simulink model "mpu6050 - Copy"  (R2017a)
settings: Solver=FixedStepDiscrete  StartTime=0.0  StopTime=inf  RelTol=1e-3
PostLoadFcn:
  | ChipSelect = 1;  % choose I2C comms
  | AddressAlt = 0;  % use default address
  | 
  | if AddressAlt == 1
  | % b1101001 (pin AD0 is logic high).
  | SlvAddr = uint8(bin2dec('1101001'));  % ADDR ALT = 1
  | else
  | % b1101000 (pin AD0 is logic low)
  | SlvAddr = uint8(bin2dec('1101000'));  % ADDR ALT = 0
  | end
  | SlvAddr = uint8(hex2dec('68'));
  | 
  | 
  | % 0x3B 59 ACCEL_XOUT[15:8]
  | % 0x3C 60 ACCEL_XOUT[7:0]
  | % 0x3D 61 ACCEL_YOUT[15:8]
  | % 0x3E 62 ACCEL_YOUT[7:0]
  | % 0x3F 63 ACCEL_ZOUT[15:8]
  | % 0x40 64 ACCEL_ZOUT[7:0]
  | 
  | AccelXRegAddr = uint8(hex2dec('3B'));
  | AccelYRegAddr = uint8(hex2dec('3D'));
  | AccelZRegAddr = uint8(hex2dec('3F'));
  | 
  | % 0x43 67 GYRO_XOUT[15:8]
  | % 0x44 68 GYRO_XOUT[7:0]
  | % 0x45 69 GYRO_YOUT[15:8]
  | % 0x46 70 GYRO_YOUT[7:0]
  | % 0x47 71 GYRO_ZOUT[15:8]
  | % 0x48 72 GYRO_ZOUT[7:0]
  | 
  | GyroXRegAddr = uint8(hex2dec('43'));
  | GyroYRegAddr = uint8(hex2dec('45'));
  | GyroZRegAddr = uint8(hex2dec('47'));
  | 
  | deviceAddr = fi(SlvAddr,0,7,0);
  | 
  | powerRegAddr = uint8(hex2dec('6B'));
  | powerRegData = bin2dec('10000001');
(part 4 of 4)

== stateflow chart mpu6050 - Copy/I2C_MPU6050_IP/MPU6050_Interface2 ==
  settings: executeAtInitialization=1
  note: I2C Configuration for MPU6050
  state init
    %initstate
    Valid_Out = 0;
    isDeviceSetup = 0;
    slv_addr = SlvAddr;
    %TODO delete all
    tmp = 0;
    tmpConfig = 0;
    tmpReadGyro = 0;
    tmpReadAccel = 0;
    tmpValid = 0;
    tmpReadDevice = 0;
    tmpHere = 0;
    tmpData = 128;
    gyroRes = 250.0/32768.0;
    accelRes = 2.0/32768.0;
  note: 0x3B 59 ACCEL_XOUT[15:8]
      | 0x3C 60 ACCEL_XOUT[7:0]
      | 0x3D 61 ACCEL_YOUT[15:8]
      | 0x3E 62 ACCEL_YOUT[7:0]
      | 0x3F 63 ACCEL_ZOUT[15:8]
      | 0x40 64 ACCEL_ZOUT[7:0]
      |
      | 0x43 67 GYRO_XOUT[15:8]
      | 0x44 68 GYRO_XOUT[7:0]
      | 0x45 69 GYRO_YOUT[15:8]
      | 0x46 70 GYRO_YOUT[7:0]
      | 0x47 71 GYRO_ZOUT[15:8]
      | 0x48 72 GYRO_ZOUT[7:0]
      |
      | 0x6B 107 PWR_MGMT_1
      | 0x6C 108 PWR_MGMT_2
  note: TODO check functions - dont need to convert?
  state idle
    %idlestate
    enb 	= 0;
    rw 		= 0;
    mode 	= 0;
    cnt      = 0;
    reg_byte_mode = 0;
    tmp = isDeviceSetup;
  state Configuration [group]
    state configurationStart
      %force success config
      isDeviceSetup = 0;
    state setupReadWhoAmI
      entry:
      enb = 1;
      rw = 1;
      mode = 0;
      reg_addr = 117;
    state waitforNotBusy0
      enb=0; tmpData=1;
    state readWhoAmI1
      %tmpData = uint8(data_in);
    state setupReadPwrMgmt1
      entry:
      enb = 1;
      rw = 1;
      mode = 0;
      reg_addr = 107;
    state waitforNotBusy1
      enb=0; tmpData=2;
    state setupWritePwrMgmt1
      enb = 1;
      rw = 0;
      mode = 0;
      reg_addr = 107; %0x6B
      data_out = 0;
    state readPwrManagement1
      tmpData = uint8(data_in);
    state waitforNotBusy2
      enb=0; %tmpData=3;
    state setupFS_SEL
      enb = 1;
      rw = 0;
      mode = 0;
      reg_addr = 27; %0x1b
      data_out = 16; %fs range +/- 1000
    state waitforNotBusy3
      enb=0; %tmpData=3;
    state configStartBiasLoop
      i = 0; biasSamples = 1000;
      GyroX = 0;  gyroXBias = 0;
      GyroY = 0;  gyroYBias = 0;
      GyroZ = 0;  gyroZBias = 0;
      AccelX = 0; accelXBias = 0;
      AccelY = 0; accelYBias = 0;
      AccelZ = 0; accelZBias = 0;
      gyroTmpBiasX = 0; gyroTmpBiasY = 0;
      gyroTmpBiasZ = 0;
      accelTmpBiasX = 0; accelTmpBiasY = 0;
      accelTmpBiasZ = 0;
      tmpHere = 1;
    state incrementBias
      i = sum_int16(i,1);
      accelTmpBiasX = sum_int16(accelTmpBiasX,AccelX);
      accelTmpBiasY = sum_int16(accelTmpBiasY,AccelY);
      accelTmpBiasZ = sum_int16(accelTmpBiasZ,AccelZ);
      gyroTmpBiasX  = sum_int16(gyroTmpBiasX, GyroX);
      gyroTmpBiasY  = sum_int16(gyroTmpBiasY, GyroY);
      gyroTmpBiasZ  = sum_int16(gyroTmpBiasZ, GyroZ);
    state configCalculateBiases
      accelXBias = divide_int16(accelTmpBiasX,biasSamples);
      accelYBias = divide_int16(accelTmpBiasY,biasSamples);
      %accelZBias = divide_int16(accelTmpBiasZ,biasSamples);
      gyroXBias  = divide_int16(gyroTmpBiasX, biasSamples);
      gyroYBias  = divide_int16(gyroTmpBiasY, biasSamples);
      %gyroZBias  = divide_int16(gyroTmpBiasZ, biasSamples);
    state cfgDone
      isDeviceSetup = 1;
      tmpConfig = 1;
      tmpHere = 0;
    configurationStart -> setupReadWhoAmI
    setupReadWhoAmI -> waitforNotBusy0 : [busy==1]
    waitforNotBusy0 -> readWhoAmI1 [order 2] : [mstr_ack==1]
    waitforNotBusy0 -> (junction 2445) [order 1] : [n_ack==1]
    readWhoAmI1 -> setupReadPwrMgmt1 : [busy==0]
    setupReadPwrMgmt1 -> Configuration.waitforNotBusy1 : [busy==1]
    Configuration.waitforNotBusy1 -> (junction 2445) [order 1] : [n_ack==1]
    Configuration.waitforNotBusy1 -> readPwrManagement1 [order 2] : [mstr_ack==1]
    readPwrManagement1 -> setupWritePwrMgmt1 : [busy==0]
    setupWritePwrMgmt1 -> waitforNotBusy2 : [busy==1]
    waitforNotBusy2 -> setupFS_SEL [order 1] : [busy==0]
    waitforNotBusy2 -> (junction 2445) [order 2] : [n_ack==1]
    setupFS_SEL -> waitforNotBusy3 : [busy==1]
    waitforNotBusy3 -> configStartBiasLoop : [busy==0]
    configStartBiasLoop -> incrementBias
    incrementBias -> configCalculateBiases [order 2]
    configCalculateBiases -> cfgDone
  state ReadDeviceData [group]
    note: DEVID is an example of
        | doing a 1-byte READ
    note: 0x75 117 - WHO_AM_I[6:1]
        | TODO
        |    THIS IS DEBUGGING ONLY DELETE!
    state getDEVID
      entry:
      enb = 1;
      rw = 1;
      mode = 0;
      reg_addr =   uint8(117);
      tmpReadDevice = 1;
    state waitforNotBusy1
      enb=0;
    state readDEVID
      deviceId = uint8(data_in);
    state waitforNotBusy6
      %
    state getRegData
      entry:
      enb = 1;
      rw = 1;
      mode = 0;
      reg_addr = userRegAddr;
    state waitforNotBusy5
      enb=0;
    state readUserRegData
      regdata = uint8(data_in);
    getDEVID -> ReadDeviceData.waitforNotBusy1 : [busy==1]
    ReadDeviceData.waitforNotBusy1 -> waitforNotBusy6 [order 2] : [n_ack==1]
    ReadDeviceData.waitforNotBusy1 -> readDEVID [order 1] : [mstr_ack==1]
    readDEVID -> getRegData : [busy==0]
    waitforNotBusy6 -> (junction 2281)
    getRegData -> waitforNotBusy5 : [busy==1]
    waitforNotBusy5 -> readUserRegData [order 1] : [mstr_ack==1]
    waitforNotBusy5 -> (junction 2281) [order 2] : [n_ack==1]
  state Valid
    en: enb = 0;
    cnt = 0;
    Valid_Out = 1;
    du: cnt = cnt + 1;
    tmpValid = 1;
  state check_cfg
    en: enb = 0;
    cnt = 0;
    du: cnt = cnt + 1;
    tmpCheckCng = 1
  state SetupBias [group] [commented out]
    state biasWritePwrMgmt1 [commented out]
      %reset device
      enb = 1;
      rw = 0;
      mode = 0;
      reg_addr = 107; %0x6B
      data_out = 128;
    state waitforNotBusyb [commented out]
      enb=0; i =0;
    state delay [commented out]
      i = i + 1;
    state biasWritePwrMgmt2 [commented out]
      enb = 1;
      rw = 0;
      mode = 0;
      reg_addr = 107; %0x6B
      data_out = 1;
    state waitforNotBusyb1 [commented out]
      enb=0; i =0;
    state biasWritePwrMgmt1_1 [commented out]
      enb = 1;
      rw = 0;
      mode = 0;
      reg_addr = 107; %0x6B
      data_out = 1;
    state waitforNotBusyb2 [commented out]
      enb=0; i =0;
    state delay1 [commented out]
      i = i + 1;
    state biasWriteIntEnable [commented out]
      %disable all interrupts
      enb = 1;
      rw = 0;
      mode = 0;
      reg_addr = 56;
      data_out = 00;
    state waitforNotBusyb3 [commented out]
      enb=0; i =0;
    state biasWriteFIFO [commented out]
      %disable FIFO
      enb = 1;
      rw = 0;
      mode = 0;
      reg_addr = 35;
      data_out = 00;
    state waitforNotBusyb4 [commented out]
      enb=0; i =0;
    state biasWritePwrMgmt1_2 [commented out]
      %turn on internal clk src
      enb = 1;
      rw = 0;
      mode = 0;
      reg_addr = 107;
      data_out = 00;
    state waitforNotBusyb5 [commented out]
      enb=0; i =0;
    state biasWriteI2cMstrCtrl [commented out]
      %disable i2c master
      enb = 1;
      rw = 0;
      mode = 0;
      reg_addr = 36;
      data_out = 00;
    state waitforNotBusyb6 [commented out]
      enb=0; i =0;
    state biasWriteUserCtrl [commented out]
      %disable FIFO & i2c maste
      enb = 1;
      rw = 0;
      mode = 0;
      reg_addr = 36;
      data_out = 00;
    state waitforNotBusyb7 [commented out]
      enb=0; i =0;
    state biasWriteUserCtrl1 [commented out]
      %reset FIFO & DMP
      enb = 1;
      rw = 0;
      mode = 0;
      reg_addr = 36;
      data_out = 12;
    state waitforNotBusyb8 [commented out]
      enb=0; i =0;
    state delay2 [commented out]
      i = i + 1;
    state biasWriteConfig [commented out]
      %set lowpassfilter to 188hz
      enb = 1;
      rw = 0;
      mode = 0;
      reg_addr = 26;
      data_out = 1;
    state waitforNotBusyb9 [commented out]
      enb=0; i =0;
    state biasWriteSmplrtDiv [commented out]
      %samplerate 1khz
      enb = 1;
      rw = 0;
      mode = 0;
      reg_addr = 36;
      data_out = 26;
    state waitforNotBusyb10 [commented out]
      enb=0; i =0;
    waitforNotBusyb -> (junction 2753) [commented out] : [n_ack==1]
    biasWritePwrMgmt1 -> waitforNotBusyb [commented out] : [busy==1]
    waitforNotBusyb -> delay [commented out] : [busy==0]
    delay -> delay [commented out] : [i < 100]
    delay -> biasWritePwrMgmt2 [commented out]
    waitforNotBusyb1 -> (junction 2753) [commented out] : [n_ack==1]
    biasWritePwrMgmt2 -> waitforNotBusyb1 [commented out] : [busy==1]
    waitforNotBusyb1 -> biasWritePwrMgmt1_1 [commented out] : [busy==0]
    waitforNotBusyb2 -> (junction 2753) [commented out] : [n_ack==1]
    waitforNotBusyb3 -> (junction 2753) [commented out] : [n_ack==1]
    (junction 2753) -> (junction 2832) [commented out]
    waitforNotBusyb4 -> (junction 2753) [commented out] : [n_ack==1]
    waitforNotBusyb5 -> (junction 2753) [commented out] : [n_ack==1]
    biasWritePwrMgmt1_1 -> waitforNotBusyb2 [commented out] : [busy==1]
    waitforNotBusyb2 -> delay1 [commented out] : [busy==0]
    delay1 -> biasWriteIntEnable [commented out]
    delay1 -> delay1 [commented out] : [i < 200]
    biasWriteIntEnable -> waitforNotBusyb3 [commented out] : [busy==1]
    waitforNotBusyb3 -> biasWriteFIFO [commented out] : [busy==0]
    biasWriteFIFO -> waitforNotBusyb4 [commented out] : [busy==1]
    waitforNotBusyb4 -> biasWritePwrMgmt1_2 [commented out] : [busy==0]
    biasWritePwrMgmt1_2 -> waitforNotBusyb5 [commented out] : [busy==1]
    waitforNotBusyb5 -> biasWriteI2cMstrCtrl [commented out] : [busy==0]
    waitforNotBusyb6 -> (junction 2834) [commented out] : [n_ack==1]
    waitforNotBusyb7 -> (junction 2834) [commented out] : [n_ack==1]
    waitforNotBusyb8 -> (junction 2834) [commented out] : [n_ack==1]
    (junction 2834) -> (junction 2832) [commented out]
    waitforNotBusyb9 -> (junction 2834) [commented out] : [n_ack==1]
    biasWriteI2cMstrCtrl -> waitforNotBusyb6 [commented out] : [busy==1]
    waitforNotBusyb6 -> biasWriteUserCtrl [commented out] : [busy==0]
    biasWriteUserCtrl -> waitforNotBusyb7 [commented out] : [busy==1]
    waitforNotBusyb7 -> biasWriteUserCtrl1 [commented out] : [busy==0]
    (junction 2869) -> (junction 2832) [commented out]
    biasWriteUserCtrl1 -> waitforNotBusyb8 [commented out] : [busy==1]
    waitforNotBusyb8 -> delay2 [commented out] : [busy==0]
    delay2 -> delay2 [commented out] : [i < 200]
    delay2 -> biasWriteConfig [commented out]
    biasWriteConfig -> waitforNotBusyb9 [commented out] : [busy==1]
    waitforNotBusyb9 -> biasWriteSmplrtDiv [commented out] : [busy==0]
    biasWriteSmplrtDiv -> waitforNotBusyb10 [commented out] : [busy==1]
    waitforNotBusyb10 -> (junction 2869) [commented out] : [n_ack==1]
    waitforNotBusyb10 -> ? [commented out] : [busy==0]
  state ReadAccelData [group]
    state setupReadAccelXoutH
      entry:
      enb = 1;
      rw = 1;
      mode = 0;
      reg_addr = 59; %0x3b
      tmpReadAccel = 1;
    state waitforNotBusya1
      enb=0; tmpData = 1;
    state readAccelXoutH
      tempVal = uint8(data_in);
      tmpData = 2;
    state setupReadAccelXoutL
      entry:
      enb = 1;
      rw = 1;
      mode = 0;
      reg_addr = 60; %0x3c
    state waitforNotBusya3
      enb=0; tmpData = 2;
    state readAccelXoutL
      AccelX = convert_int16(tempVal, data_in);
      AccelX = subtract_int16(AccelX,accelXBias);
    state setupReadAccelYoutH
      entry:
      enb = 1;
      rw = 1;
      mode = 0;
      reg_addr = 61; %0x3d
    state waitforNotBusya4
      enb=0; tmpData = 3;
    state readAccelYoutH
      tempVal = uint8(data_in);
    state setupReadAccelYoutL
      entry:
      enb = 1;
      rw = 1;
      mode = 0;
      reg_addr = 62; %0x3e
    state waitforNotBusya5
      enb=0;tmpData = 4;
    state readGyroYoutL
      AccelY = convert_int16(tempVal, data_in)
      AccelY = subtract_int16(AccelY,accelYBias);;
    state setupReadAccelZoutH
      entry:
      enb = 1;
      rw = 1;
      mode = 0;
      reg_addr = 63; %0x3f
    state waitforNotBusya6
      enb=0;tmpData = 5;
    state readAccelZoutH
      tempVal = uint8(data_in);
    state setupReadAccelZoutL
      entry:
      enb = 1;
      rw = 1;
      mode = 0;
      reg_addr = 64; %0x40
    state waitforNotBusya7
      enb=0;tmpData = 6;
    state readAccelZoutL
      AccelZ = convert_int16(tempVal, data_in);
      %AccelZ = subtract_int16(AccelZ,accelZBias);
    setupReadAccelXoutH -> waitforNotBusya1 : [busy==1]
    waitforNotBusya1 -> (junction 2534) [order 2] : [n_ack==1]
    waitforNotBusya1 -> readAccelXoutH [order 1] : [mstr_ack==1]
    readAccelXoutH -> setupReadAccelXoutL : [busy==0]
    setupReadAccelXoutL -> waitforNotBusya3 : [busy==1]
    waitforNotBusya3 -> (junction 2534) [order 2] : [n_ack==1]
    waitforNotBusya3 -> readAccelXoutL [order 1] : [mstr_ack==1]
    readAccelXoutL -> setupReadAccelYoutH : [busy==0]
    waitforNotBusya4 -> (junction 2534) [order 2] : [n_ack==1]
    waitforNotBusya5 -> (junction 2534) [order 2] : [n_ack==1]
    waitforNotBusya6 -> (junction 2534) [order 2] : [n_ack==1]
    waitforNotBusya7 -> (junction 2534) [order 2] : [n_ack==1]
    setupReadAccelYoutH -> waitforNotBusya4 : [busy==1]
    waitforNotBusya4 -> readAccelYoutH [order 1] : [mstr_ack==1]
    readAccelYoutH -> setupReadAccelYoutL : [busy==0]
    setupReadAccelYoutL -> waitforNotBusya5 : [busy==1]
    waitforNotBusya5 -> ReadAccelData.readGyroYoutL [order 1] : [mstr_ack==1]
    ReadAccelData.readGyroYoutL -> setupReadAccelZoutH : [busy==0]
    setupReadAccelZoutH -> waitforNotBusya6 : [busy==1]
    waitforNotBusya6 -> readAccelZoutH [order 1] : [mstr_ack==1]
    readAccelZoutH -> setupReadAccelZoutL : [busy==0]
    setupReadAccelZoutL -> waitforNotBusya7 : [busy==1]
    waitforNotBusya7 -> readAccelZoutL [order 1] : [mstr_ack==1]
  state ReadGyroData [group]
    state setupReadGyroXoutH
      entry:
      enb = 1;
      rw = 1;
      mode = 0;
      reg_addr = 67; %0x43
      tmpReadGyro = 1;
    state waitforNotBusy06
      enb=0;tmpData = 10;
    state readGyroXoutH
      tempVal = uint8(data_in);
    state setupReadGyroXoutL
      entry:
      enb = 1;
      rw = 1;
      mode = 0;
      reg_addr = 68; %0x44
    state waitforNotBusy07
      enb=0;tmpData = 11;
    state readGyroXoutL
      GyroX = convert_int16(tempVal, data_in);
      GyroX = subtract_int16(GyroX,gyroXBias);
    state setupReadGyroYoutH
      entry:
      enb = 1;
      rw = 1;
      mode = 0;
      reg_addr = 69; %0x45
    state waitforNotBusy04
      enb=0;tmpData = 12;
    state readGyroYoutH
      tempVal = uint8(data_in);
    state setupReadGyroYoutL
      entry:
      enb = 1;
      rw = 1;
      mode = 0;
      reg_addr = 70; %0x46
    state waitforNotBusy05
      enb=0;tmpData = 13;
    state readGyroYoutL
      GyroY = convert_int16(tempVal, data_in);
      GyroY = subtract_int16(GyroY,gyroYBias);
    state setupReadGyroZoutH
      entry:
      enb = 1;
      rw = 1;
      mode = 0;
      reg_addr = 71; %0x47
    state waitforNotBusy01
      enb=0;tmpData = 14;
    state readGyroZoutH
      tempVal = uint8(data_in);
    state setupReadGyroZoutL
      entry:
      enb = 1;
      rw = 1;
      mode = 0;
      reg_addr = 72; %0x48
    state waitforNotBusy03
      enb=0;tmpData = 15;
    state readGyroZoutL
      GyroZ = convert_int16(tempVal, data_in);
      %GyroZ = subtract_int16(GyroZ,gyroZBias);
    setupReadGyroXoutH -> waitforNotBusy06 : [busy==1]
    waitforNotBusy06 -> (junction 2595) [order 2] : [n_ack==1]
    waitforNotBusy06 -> readGyroXoutH [order 1] : [mstr_ack==1]
    readGyroXoutH -> setupReadGyroXoutL : [busy==0]
    setupReadGyroXoutL -> waitforNotBusy07 : [busy==1]
    waitforNotBusy07 -> (junction 2595) [order 2] : [n_ack==1]
    waitforNotBusy07 -> readGyroXoutL [order 1] : [mstr_ack==1]
    readGyroXoutL -> setupReadGyroYoutH : [busy==0]
    waitforNotBusy04 -> (junction 2595) [order 2] : [n_ack==1]
    waitforNotBusy05 -> (junction 2595) [order 2] : [n_ack==1]
    waitforNotBusy01 -> (junction 2595) [order 2] : [n_ack==1]
    waitforNotBusy03 -> (junction 2595) [order 2] : [n_ack==1]
    setupReadGyroYoutH -> waitforNotBusy04 : [busy==1]
    waitforNotBusy04 -> readGyroYoutH [order 1] : [mstr_ack==1]
    readGyroYoutH -> setupReadGyroYoutL : [busy==0]
    setupReadGyroYoutL -> waitforNotBusy05 : [busy==1]
    waitforNotBusy05 -> ReadGyroData.readGyroYoutL [order 1] : [mstr_ack==1]
    ReadGyroData.readGyroYoutL -> setupReadGyroZoutH : [busy==0]
    setupReadGyroZoutH -> waitforNotBusy01 : [busy==1]
    waitforNotBusy01 -> readGyroZoutH [order 1] : [mstr_ack==1]
    readGyroZoutH -> setupReadGyroZoutL : [busy==0]
    setupReadGyroZoutL -> waitforNotBusy03 : [busy==1]
    waitforNotBusy03 -> readGyroZoutL [order 1] : [mstr_ack==1]
    readGyroZoutL -> (junction 2952) : [busy==0]
  note: https://github.com/kriswiner/MPU6050/blob/master/MPU6050BasicExample.ino
      | # define GYRO_CONFIG 0x1B
      | #define ACCEL_CONFIG 0x1C
      | gRes = 250.0/32768.0;
      | aRes = 2.0/32768.0;
      | ///////////////////////////////////////////////////////////////////////////////////////////////////////////END calibrate/////////////////////////////////////////////////////////////////////////////////////////////
      | // reset device, reset all registers, clear gyro and accelerometer bias registers
      | writeByte(MPU6050_ADDRESS, PWR_MGMT_1, 0x80); // Write a one to bit 7 reset bit; toggle reset device
      | delay(100);
      |
      | // get stable time source
      | // Set clock source to be PLL with x-axis gyroscope reference, bits 2:0 = 001
      | writeByte(MPU6050_ADDRESS, PWR_MGMT_1, 0x01);
      | writeByte(MPU6050_ADDRESS, PWR_MGMT_2, 0x00);
      | delay(200);
      | // Configure device for bias calculation
      | writeByte(MPU6050_ADDRESS, INT_ENABLE, 0x00); // Disable all interrupts
      | writeByte(MPU6050_ADDRESS, FIFO_EN, 0x00); // Disable FIFO
      | writeByte(MPU6050_ADDRESS, PWR_MGMT_1, 0x00); // Turn on internal clock source
      | writeByte(MPU6050_ADDRESS, I2C_MST_CTRL, 0x00); // Disable I2C master
      | writeByte(MPU6050_ADDRESS, USER_CTRL, 0x00); // Disable FIFO and I2C master modes
      | writeByte(MPU6050_ADDRESS, USER_CTRL, 0x0C); // Reset FIFO and DMP
      | delay(15);
      | // Configure MPU6050 gyro and accelerometer for bias calculation
      | writeByte(MPU6050_ADDRESS, CONFIG, 0x01); // Set low-pass filter to 188 Hz
      | writeByte(MPU6050_ADDRESS, SMPLRT_DIV, 0x00); // Set sample rate to 1 kHz
      | writeByte(MPU6050_ADDRESS, GYRO_CONFIG, 0x00); // Set gyro full-scale to 250 degrees per second, maximum sensitivity
      | writeByte(MPU6050_ADDRESS, ACCEL_CONFIG, 0x00); // Set accelerometer full-scale to 2 g, maximum sensitivity
      | uint16_t gyrosensitivity = 131; // = 131 LSB/degrees/sec
      | uint16_t accelsensitivity = 16384; // = 16384 LSB/g
      | // Configure FIFO to capture accelerometer and gyro data for bias calculation
      | writeByte(MPU6050_ADDRESS, USER_CTRL, 0x40); // Enable FIFO
      | writeByte(MPU6050_ADDRESS, FIFO_EN, 0x78); // Enable gyro and accelerometer sensors for FIFO (max size 1024 bytes in MPU-6050)
      | delay(80); // accumulate 80 samples in 80 milliseconds = 960 bytes
      | // At end of sample accumulation, turn off FIFO sensor read
      | writeByte(MPU6050_ADDRESS, FIFO_EN, 0x00); // Disable gyro and accelerometer sensors for FIFO
      | readBytes(MPU6050_ADDRESS, FIFO_COUNTH, 2, &data[0]); // read FIFO sample count
      | fifo_count = ((uint16_t)data[0] << 8) | data[1];
      | packet_count = fifo_count/12;// How many sets of full gyro and accelerometer data for averaging
      | for (ii = 0; ii < packet_count; ii++) {
      | int16_t accel_temp[3] = {0, 0, 0}, gyro_temp[3] = {0, 0, 0};
      | readBytes(MPU6050_ADDRESS, FIFO_R_W, 12, &data[0]); // read data for averaging
      | accel_temp[0] = (int16_t) (((int16_t)data[0] << 8) | data[1] ) ; // Form signed 16-bit integer for each sample in FIFO
      | accel_temp[1] = (int16_t) (((int16_t)data[2] << 8) | data[3] ) ;
      | accel_temp[2] = (int16_t) (((int16_t)data[4] << 8) | data[5] ) ;
      | gyro_temp[0] = (int16_t) (((int16_t)data[6] << 8) | data[7] ) ;
      | gyro_temp[1] = (int16_t) (((int16_t)data[8] << 8) | data[9] ) ;
      | gyro_temp[2] = (int16_t) (((int16_t)data[10] << 8) | data[11]) ;
      |
      | accel_bias[0] += (int32_t) accel_temp[0]; // Sum individual signed 16-bit biases to get accumulated signed 32-bit biases
      | accel_bias[1] += (int32_t) accel_temp[1];
      | accel_bias[2] += (int32_t) accel_temp[2];
      | gyro_bias[0] += (int32_t) gyro_temp[0];
      | gyro_bias[1] += (int32_t) gyro_temp[1];
      | gyro_bias[2] += (int32_t) gyro_temp[2];
      |
      | }
      | accel_bias[0] /= (int32_t) packet_count; // Normalize sums to get average count biases
      | accel_bias[1] /= (int32_t) packet_count;
      | accel_bias[2] /= (int32_t) packet_count;
      | gyro_bias[0] /= (int32_t) packet_count;
      | gyro_bias[1] /= (int32_t) packet_count;
      | gyro_bias[2] /= (int32_t) packet_count;
      |
      | if(accel_bias[2] > 0L) {accel_bias[2] -= (int32_t) accelsensitivity;} // Remove gravity from the z-axis accelerometer bias calculation
      | else {accel_bias[2] += (int32_t) accelsensitivity;}
      |
      | // Construct the gyro biases for push to the hardware gyro bias registers, which are reset to zero upon device startup
      | data[0] = (-gyro_bias[0]/4 >> 8) & 0xFF; // Divide by 4 to get 32.9 LSB per deg/s to conform to expected bias input format
      | data[1] = (-gyro_bias[0]/4) & 0xFF; // Biases are additive, so change sign on calculated average gyro biases
      | data[2] = (-gyro_bias[1]/4 >> 8) & 0xFF;
      | data[3] = (-gyro_bias[1]/4) & 0xFF;
      | data[4] = (-gyro_bias[2]/4 >> 8) & 0xFF;
      | data[5] = (-gyro_bias[2]/4) & 0xFF;
      |
      | // Push gyro biases to hardware registers; works well for gyro but not for accelerometer
      | // writeByte(MPU6050_ADDRESS, XG_OFFS_USRH, data[0]);
      | // writeByte(MPU6050_ADDRESS, XG_OFFS_USRL, data[1]);
      | // writeByte(MPU6050_ADDRESS, YG_OFFS_USRH, data[2]);
      | // writeByte(MPU6050_ADDRESS, YG_OFFS_USRL, data[3]);
      | // writeByte(MPU6050_ADDRESS, ZG_OFFS_USRH, data[4]);
      | // writeByte(MPU6050_ADDRESS, ZG_OFFS_USRL, data[5]);
      |
      | dest1[0] = (float) gyro_bias[0]/(float) gyrosensitivity; // construct gyro bias in deg/s for later manual subtraction
      | dest1[1] = (float) gyro_bias[1]/(float) gyrosensitivity;
      | dest1[2] = (float) gyro_bias[2]/(float) gyrosensitivity;
      | ///////////////////////////////////////////////////////////////////////////////////////////////////////////END calibrate/////////////////////////////////////////////////////////////////////////////////////////////
      | writeByte(MPU6050_ADDRESS, PWR_MGMT_1, 0x80); // Write a one to bit 7 reset bit; toggle reset device
      | delay(100);
      | init();
      |
      | readAccelData(accelCount); // Read the x/y/z adc values
      | getAres();
      |
      | // Now we'll calculate the accleration value into actual g's
      | ax = (float)accelCount[0]*aRes - accelBias[0]; // get actual g value, this depends on scale being set
      | ay = (float)accelCount[1]*aRes - accelBias[1];
      | az = (float)accelCount[2]*aRes - accelBias[2];
      |
      | readGyroData(gyroCount); // Read the x/y/z adc values
      | getGres();
      |
      | // Calculate the gyro value into actual degrees per second
      | gx = (float)gyroCount[0]*gRes - gyroBias[0]; // get actual gyro value, this depends on scale being set
      | gy = (float)gyroCount[1]*gRes - gyroBias[1];
      | gz = (float)gyroCount[2]*gRes - gyroBias[2];
  (default) -> init
  init -> idle
  check_cfg -> idle : [cnt >=5]
  (junction 2460) -> configurationStart [order 1] : [configDevice==1 | isDeviceSetup == 0]
  idle -> (junction 2460) : [busy==0]
  (junction 2460) -> getDEVID [order 2]
  (junction 2445) -> check_cfg
  readUserRegData -> setupReadAccelXoutH : [busy==0]
  (junction 2281) -> check_cfg
  Valid -> check_cfg : [cnt >= 5]
  (junction 2595) -> check_cfg
  (junction 2534) -> check_cfg
  (junction 2952) -> Valid [order 2]
  incrementBias -> setupReadAccelXoutH [order 1] : [i<biasSamples]
  (junction 2952) -> incrementBias [order 1] : [isDeviceSetup==0]
  readAccelZoutL -> setupReadGyroXoutH : [busy==0]
  cfgDone -> setupReadAccelXoutH
  data: a function_input uint8; b function_input uint8; val function_output int16; a function_input uint8; b function_input uint8; val function_output int16; msb function_input uint8; lsb function_input uint8; val function_output int16; a function_input uint8; b function_input uint8; val function_output int16; enb output boolean size=1; rw output boolean size=1; mode output boolean; slv_addr output uint8; reg_addr output uint8; reg_byte_mode output boolean size=1; data_out output uint8; busy input; n_ack input; byte_mode input boolean size=1; reg_mode input boolean size=1; cnt local uint32; data_in input uint8 size=1; mstr_ack input; AccelX output int16; AccelY output int16; AccelZ output int16; SlvAddr parameter uint8; Valid_Out output boolean; tempVal local uint8; deviceId output uint8; regdata output uint8; userRegAddr input uint8; configDevice input boolean; GyroX output int16; GyroY output int16; GyroZ output int16; tmp output boolean; tmpConfig output boolean; tmpCheckCng output boolean; tmpReadGyro output boolean; tmpReadAccel output boolean; tmpValid output boolean; tmpReadDevice output boolean; tmpHere output boolean; tmpData output uint8; accelRes local double; gyroRes local double; i local int16; isDeviceSetup output boolean; accelXBias output int16; biasSamples local int16; accelYBias output int16; accelZBias output int16; gyroXBias output int16; gyroYBias output int16; gyroZBias output int16; gyroTmpBiasX local int16; gyroTmpBiasY local int16; gyroTmpBiasZ local int16; accelTmpBiasX local int16; accelTmpBiasY local int16; accelTmpBiasZ local int16
  function val = sum_int16(a,b):
    | function val = sum_int16(a,b)
    |     %val = int16(a+b);
    |     val = int16(a+b);
  function val = subtract_int16(a,b):
    | function val = subtract_int16(a,b)
    |     %val = int16(a-b);
    |     val = int16(a-b);
  function val = convert_int16(msb, lsb):
    | function val = convert_int16(msb, lsb)
    | 
    | val = int16(bitor(bitshift(int16(msb),8), int16(lsb)));
  function val = divide_int16(a,b):
    | function val = divide_int16(a,b)
    |     %val = int16(a/b);
    |     val = int16(a/b);
